simulink model "Error_Performance_Indexes"  (R2020a)
settings: Solver=FixedStepAuto  StartTime=0.0  StopTime=15  FixedStep=0.001  RelTol=1e-3
settings Model: Creator=Sergio  LastModifiedBy=Sergio

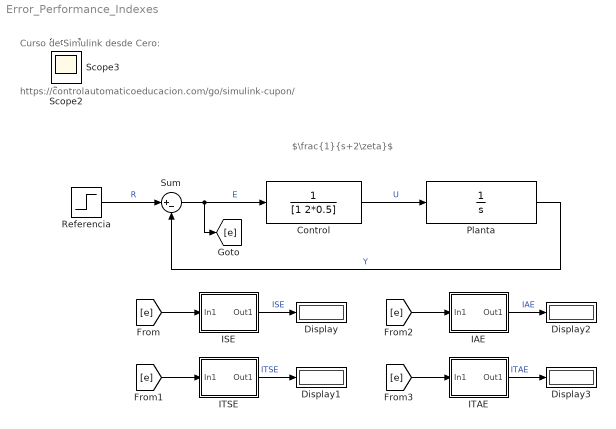
== system Error_Performance_Indexes ==
  note: $\frac{1}{s+2\zeta}$
  note: https://controlautomaticoeducacion.com/go/simulink-cupon/
  note: Curso de Simulink desde Cero:
  Control : TransferFcn  Denominator=[1 2*0.5]
  Display{,1..3} (4 alike) : Display
  IAE : Subsystem
  ISE : Subsystem
  ITAE : Subsystem
  ITSE : Subsystem
  Planta : TransferFcn  Denominator=[1 0]
  Referencia : Step  Time=0  SampleTime=0
  Sum : Sum  Inputs=|+-
  Scope{,1..3} (4 alike) : Scope
  wires:
  Referencia/1 -> Sum/1  "R"
  Sum/1 -> Control/1, [e]  "E"
  Control/1 -> Planta/1  "U"
  Planta/1 -> Sum/2  "Y"
  [e] -> ISE/1(In1)
  ISE/1(Out1) -> Display/1  "ISE"
  ITSE/1(Out1) -> Display1/1  "ITSE"
  [e] -> ITSE/1(In1)
  [e] -> IAE/1(In1)
  IAE/1(Out1) -> Display2/1  "IAE"
  ITAE/1(Out1) -> Display3/1  "ITAE"
  [e] -> ITAE/1(In1)

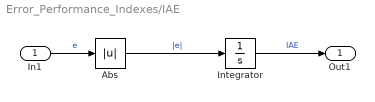
== system Error_Performance_Indexes/IAE ==
  In1 : Inport
  Abs : Abs
  Integrator : Integrator
  Out1 : Outport
  wires:
  Integrator/1 -> Out1/1  "IAE"
  In1/1 -> Abs/1  "e"
  Abs/1 -> Integrator/1  "|e|"

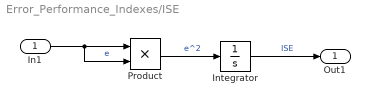
== system Error_Performance_Indexes/ISE ==
  In1 : Inport
  Integrator : Integrator
  Product : Product
  Out1 : Outport
  wires:
  In1/1 -> Product/2, Product/1  "e"
  Product/1 -> Integrator/1  "e^2"
  Integrator/1 -> Out1/1  "ISE"

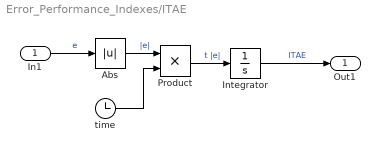
== system Error_Performance_Indexes/ITAE ==
  In1 : Inport
  Abs : Abs
  Integrator : Integrator
  Product : Product
  time : Clock
  Out1 : Outport
  wires:
  In1/1 -> Abs/1  "e"
  Integrator/1 -> Out1/1  "ITAE"
  time/1 -> Product/2
  Abs/1 -> Product/1  "|e|"
  Product/1 -> Integrator/1  "t |e|"

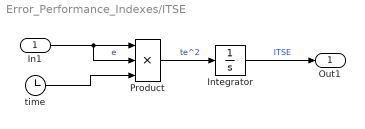
== system Error_Performance_Indexes/ITSE ==
  In1 : Inport
  Integrator : Integrator
  Product : Product  Inputs=3
  time : Clock
  Out1 : Outport
  wires:
  Integrator/1 -> Out1/1  "ITSE"
  In1/1 -> Product/1, Product/2  "e"
  time/1 -> Product/3
  Product/1 -> Integrator/1  "te^2"
